simulink model "cruise_ctrl"  (R2020a)
settings: Solver=VariableStepAuto  StartTime=0.0  StopTime=10.0  RelTol=1e-3
values from neighbouring files (symbols this model uses):
  b = 50.0    [cruise.sldd]
  kd = 50.0    [cruise.sldd]
  ki = 300.0    [cruise.sldd]
  kp = 350.0    [cruise.sldd]
  m = 1000.0    [cruise.sldd]
settings Model: DataDictionary=cruise.sldd  Creator=Shubham  LastModifiedBy=Shubham

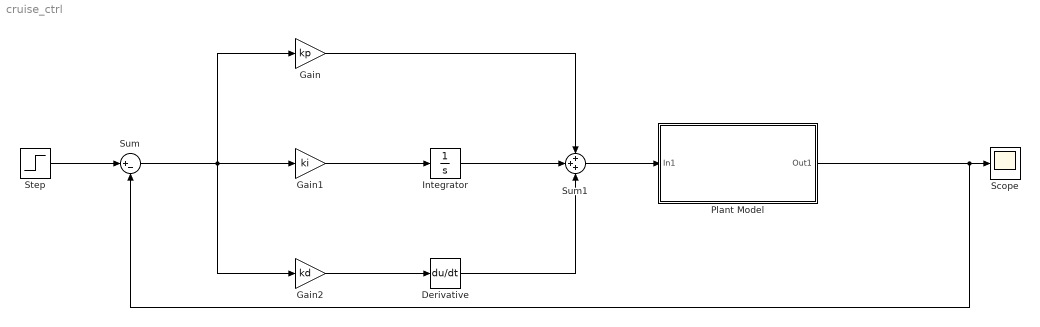
== system cruise_ctrl ==
  Derivative : Derivative
  Gain : Gain  Gain=kp
  Gain1 : Gain  Gain=ki
  Gain2 : Gain  Gain=kd
  Integrator : Integrator
  Plant Model : Subsystem
  Scope : Scope
  Step : Step  Time=0  After=u  SampleTime=0
  Sum : Sum  Inputs=|+-
  Sum1 : Sum  Inputs=+++
  wires:
  Step/1 -> Sum/1
  Sum/1 -> Gain2/1, Gain/1, Gain1/1
  Gain1/1 -> Integrator/1
  Gain2/1 -> Derivative/1
  Integrator/1 -> Sum1/2
  Gain/1 -> Sum1/1
  Derivative/1 -> Sum1/3
  Plant Model/1(Out1) -> Sum/2, Scope/1
  Sum1/1 -> Plant Model/1(In1)

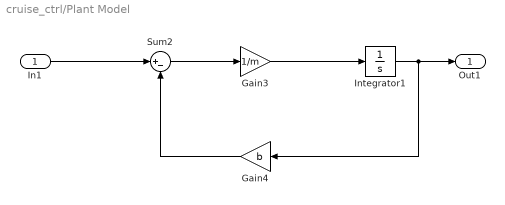
== system cruise_ctrl/Plant Model ==
  In1 : Inport
  Gain3 : Gain  Gain=1/m
  Gain4 : Gain  Gain=b
  Integrator1 : Integrator
  Sum2 : Sum  Inputs=|+-
  Out1 : Outport
  wires:
  Gain4/1 -> Sum2/2
  Integrator1/1 -> Out1/1, Gain4/1
  Gain3/1 -> Integrator1/1
  Sum2/1 -> Gain3/1
  In1/1 -> Sum2/1
